simulink model "bpsk"  (R2021b)
settings: Solver=VariableStepAuto  StartTime=0.0  StopTime=10.0  RelTol=1e-3
libraries: commrandsrc3 x1
settings Model: Creator=Leon8dem1god  LastModifiedBy=Leon8dem1god

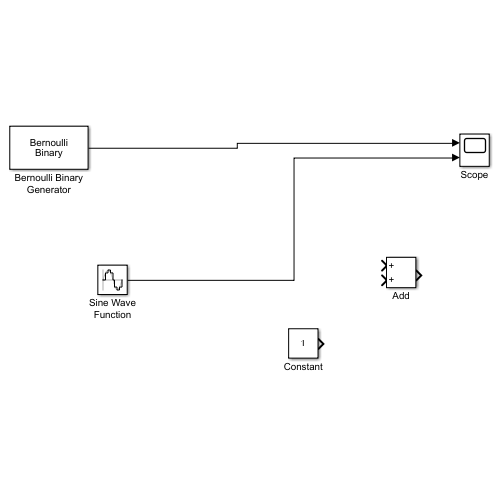
[thumbnail: Simulink's stored preview of the top-level diagram]
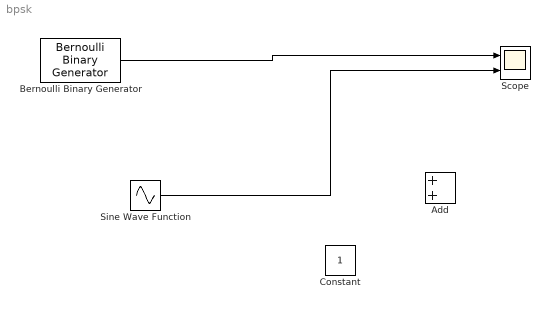
== system bpsk ==
  Add : Sum
  Bernoulli Binary Generator : commrandsrc3/Bernoulli Binary Generator  ProbabilityOfZero=0.5  SeedSource=Auto  Seed=0  SampleTime=1  SamplesPerFrame=1  OutputDataType=double  SimulateUsing=Interpreted execution
  Constant : Constant
  Scope : Scope  NumInputPorts=2
  Sine Wave Function : Sin  Frequency=4*pi  SampleTime=1/3200*pi
  wires:
  Sine Wave Function/1 -> Scope/2
  Bernoulli Binary Generator/1 -> Scope/1
